simulink model "product_matrix_multiple_test_tmp"  (Simulink 8.3)
settings: Solver=ode45  StartTime=0.0  StopTime=10.0  RelTol=1e-3
settings Model: Creator=arnaud  LastModifiedBy=hbourbou
settings DataIOCC: SaveFormat=Structure
settings OptimizationCC: ExpressionDepthLimit=2147483647
settings DebuggingCC: FcnCallInpInsideContextMsg=EnableAllAsWarning  FrameProcessingCompatibilityMsg=error

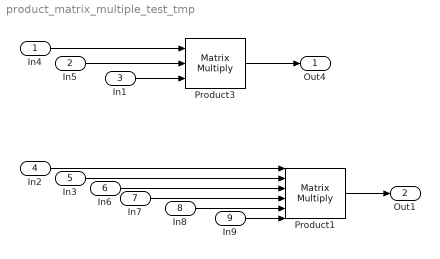
== system product_matrix_multiple_test_tmp ==
  In4 : Inport  PortDimensions=[2 3]
  In5 : Inport  Port=2  PortDimensions=[3 2]
  In1 : Inport  Port=3  PortDimensions=[2 1]
  In2 : Inport  Port=4  PortDimensions=[2 4]
  In3 : Inport  Port=5  PortDimensions=[4 2]
  In6 : Inport  Port=6  PortDimensions=[2 3]
  In7 : Inport  Port=7  PortDimensions=[3 3]
  In8 : Inport  Port=8  PortDimensions=[3 2]
  In9 : Inport  Port=9  PortDimensions=[2 1]
  Product1 : Product  Inputs=6  Multiplication=Matrix(*)  RndMeth=Zero
  Product3 : Product  Inputs=***  Multiplication=Matrix(*)  RndMeth=Zero
  Out4 : Outport
  Out1 : Outport  Port=2
  wires:
  In4/1 -> Product3/1
  Product3/1 -> Out4/1
  In5/1 -> Product3/2
  In1/1 -> Product3/3
  In2/1 -> Product1/1
  Product1/1 -> Out1/1
  In3/1 -> Product1/2
  In6/1 -> Product1/3
  In7/1 -> Product1/4
  In8/1 -> Product1/5
  In9/1 -> Product1/6
